simulink model "csu_gpe_ground_point_extraction_hrn"  (R2014b)
settings: Solver=FixedStepDiscrete  StartTime=0  StopTime=1  FixedStep=1  RelTol=1e-3
values from neighbouring files (symbols this model uses):
  camera_pose_P = cam_intrinsic_matrix_c * camera_pose_C    [csu_gpe_ground_point_extraction_test.m]
undefined symbols (not defined in the file or in its folder): corners_in, csu_gpe_ground_point_extraction, csu_gpe_ground_point_extraction_lib
settings Model: Creator=escrane  LastModifiedBy=mstewart
settings DataIOCC: SignalLoggingSaveFormat=ModelDataLogs
settings OptimizationCC: ExpressionDepthLimit=2147483647
settings DebuggingCC: UnderspecifiedInitializationDetection=Classic  MergeDetectMultiDrivingBlocksExec=none  FcnCallInpInsideContextMsg=EnableAllAsWarning  StateNameClashWarn=warning

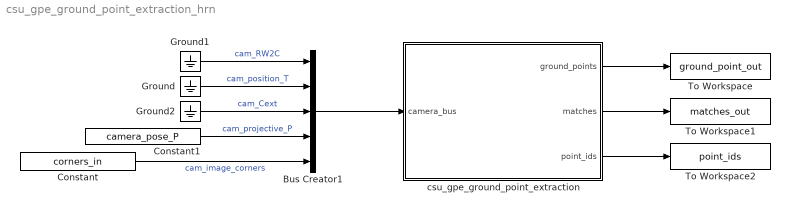
== system csu_gpe_ground_point_extraction_hrn ==
  Bus Creator1 : BusCreator  Inputs=5
  Constant : Constant  Value=corners_in
  Constant1 : Constant  Value=camera_pose_P
  Ground : Ground
  Ground1 : Ground
  Ground2 : Ground
  To Workspace : ToWorkspace  VariableName=ground_point_out  SaveFormat=Timeseries  SampleTime=-1
  To Workspace1 : ToWorkspace  VariableName=matches_out  SaveFormat=Timeseries  SampleTime=-1
  To Workspace2 : ToWorkspace  VariableName=point_ids  SaveFormat=Timeseries  SampleTime=-1
  csu_gpe_ground_point_extraction : Subsystem  AncestorBlock=csu_gpe_ground_point_extraction_lib/csu_gpe_ground_point_extraction
  wires:
  Constant/1 -> Bus Creator1/5  "cam_image_corners"
  csu_gpe_ground_point_extraction/1(ground_points) -> To Workspace/1
  Ground1/1 -> Bus Creator1/1  "cam_RW2C"
  Constant1/1 -> Bus Creator1/4  "cam_projective_P"
  Ground/1 -> Bus Creator1/2  "cam_position_T"
  Ground2/1 -> Bus Creator1/3  "cam_Cext"
  Bus Creator1/1 -> csu_gpe_ground_point_extraction/1(camera_bus)
  csu_gpe_ground_point_extraction/2(matches) -> To Workspace1/1
  csu_gpe_ground_point_extraction/3(point_ids) -> To Workspace2/1

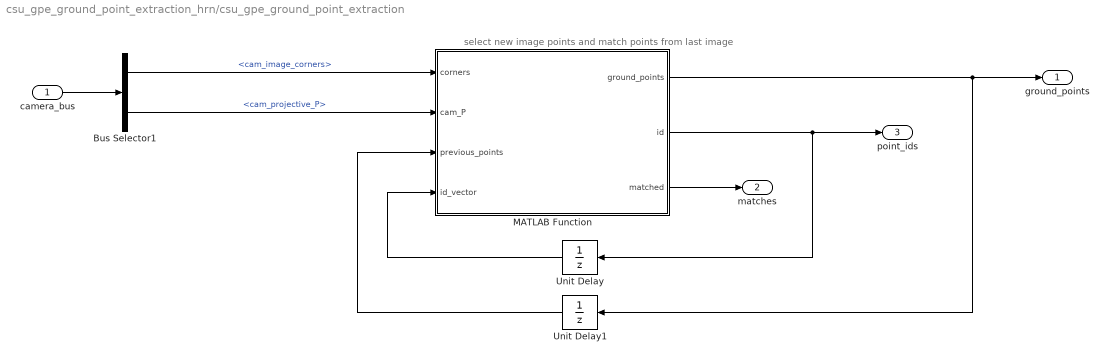
== system csu_gpe_ground_point_extraction_hrn/csu_gpe_ground_point_extraction ==
  note: select new image points and match points from last image
  camera_bus : Inport
  Bus Selector1 : BusSelector  OutputSignals=cam_image_corners,cam_projective_P
  MATLAB Function : MATLAB Function  TreatAsAtomicUnit=on
  Unit Delay : UnitDelay  InitialCondition=zeros(10,1)  SampleTime=-1
  Unit Delay1 : UnitDelay  InitialCondition=zeros(10,2)  SampleTime=-1
  ground_points : Outport
  matches : Outport  Port=2
  point_ids : Outport  Port=3
  wires:
  Unit Delay1/1 -> MATLAB Function/3(previous_points)
  Unit Delay/1 -> MATLAB Function/4(id_vector)
  MATLAB Function/2(id) -> Unit Delay/1, point_ids/1
  Bus Selector1/1 -> MATLAB Function/1(corners)  "<cam_image_corners>"
  MATLAB Function/1(ground_points) -> Unit Delay1/1, ground_points/1
  camera_bus/1 -> Bus Selector1/1
  MATLAB Function/3(matched) -> matches/1
  Bus Selector1/2 -> MATLAB Function/2(cam_P)  "<cam_projective_P>"

== matlab function csu_gpe_ground_point_extraction_hrn/csu_gpe_ground_point_extraction/MATLAB Function ==
  data: corners input double size=[4 3]; cam_P input; ground_points output double size=[10 2]; previous_points input double size=[10 2]; id_vector input double size=[10 1]; id output double size=[10 1]; matched output double size=[10 1]
function [ground_points,id,matched] = ground_point_database(corners, cam_P, previous_points, id_vector)
%#codegen

ground_points = [previous_points(6:10,:) ; zeros(5,3)];
id  = [id_vector(6:10); zeros(5,1)];
matched = zeros(10,1);

% find new points in current image (points 6:10)
new_ground_points = zeros(5,2);

% center point:
    mid_point = [mean(corners(:,1))  mean(corners(:,2))];
    new_ground_points(1,:) = mid_point;
    
% mid/corner points
    for jj = 1 : 4
        
        b = corners(jj,1:2) - mid_point;
        b = b/norm(b);
        new_ground_points(1+jj,:) = mid_point + norm(corners(jj,1:2) - mid_point)/2*b ;
         
    end

ground_points(6:10,:) = new_ground_points;
id(6:10,:) = id(5) + [1:5]';

% see if we can match points from previous image (points 1:5)
for kk = 1 : 5

        h = cam_P * [ground_points(kk,1) ; ground_points(kk,2) ; 0; 1];
        pix = h(1:2) ./ h(3);
        pix = round( pix );
        
        if ( pix(1) > 0 && pix(1) <= 640) && ( pix(2) > 0 && pix(2) <= 480) 
    
            matched(kk) = 1;    
            
        end
        
end
